simulink model "BlockModel"  (R2018b)
settings: Solver=ode45  StartTime=0.0  StopTime=10.0  RelTol=1e-3  EnableMultiTasking=on
PreLoadFcn:
  | load Buses
libraries: CustomLibrary x3
settings Model: Creator=Rose  LastModifiedBy=Rose
settings DataIOCC: LimitDataPoints=on  SaveFormat=Array  SignalLoggingSaveFormat=ModelDataLogs
settings OptimizationCC: DefaultParameterBehavior=Inlined  ExpressionDepthLimit=2147483647  LifeSpan=inf
settings DebuggingCC: UnderspecifiedInitializationDetection=Classic  MergeDetectMultiDrivingBlocksExec=none  SolverPrmCheckMsg=warning  FcnCallInpInsideContextMsg=warning  AllowSymbolicDim=off  StateNameClashWarn=warning  LibraryContextMissingDiagnostic=none  SFUnexpectedBacktrackingDiag=warning  SFNoUnconditionalDefaultTransitionDiag=warning  SFExecutionAtInitializationDiag=none
settings HardwareCC: ProdBitPerPointer=32  ProdBitPerSizeT=32  ProdBitPerPtrDiffT=32  ProdLargestAtomicFloat=None  ProdIntDivRoundTo=Undefined  ProdEndianess=Unspecified  ProdWordSize=32  ProdHWDeviceType=32-bit Generic
settings ModelReferenceCC: PropagateSignalLabelsOutOfModel=off
settings SFSimCC: SimUseLocalCustomCode=off
settings RTWCC: RTWUseLocalCustomCode=off
settings CodeAppCC: StateflowObjectComments=on
settings GRTTargetCC: TargetLangStandard=C89/C90 (ANSI)  GeneratePreprocessorConditionals=Disable all  CombineOutputUpdateFcns=off  GRTInterface=on
settings ConfigComp: CovMetricSettings=dw  CovHtmlReporting=on  CovSaveCumulativeToWorkspaceVar=on  CovSaveSingleToWorkspaceVar=on  CovExternalEMLEnable=off

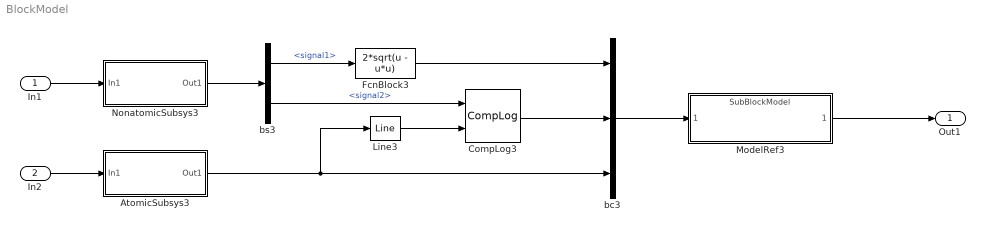
== system BlockModel ==
  In1 : Inport  OutDataTypeStr=Bus: Bus_2
  In2 : Inport  Port=2  OutDataTypeStr=int32  SampleTime=[0,1]
  AtomicSubsys3 : Subsystem  TreatAsAtomicUnit=on
  CompLog3 : CustomLibrary/CompLog  SystemSampleTime=-1
  FcnBlock3 : Fcn  Expr=2*sqrt(u - u*u)
  Line3 : CustomLibrary/Line  m=3  b=-1
  ModelRef3 : ModelReference  ModelNameDialog=SubBlockModel  SimulationMode=Normal  ModelReferenceVersion=1.41
  NonatomicSubsys3 : Subsystem
  bc3 : BusCreator  Inputs=3  OutDataTypeStr=Bus: Bus_2
  bs3 : BusSelector  OutputSignals=signal1,signal2
  Out1 : Outport  OutDataTypeStr=Bus: Bus_1
  wires:
  In1/1 -> NonatomicSubsys3/1(In1)
  In2/1 -> AtomicSubsys3/1(In1)
  NonatomicSubsys3/1(Out1) -> bs3/1
  bc3/1 -> ModelRef3/1
  AtomicSubsys3/1(Out1) -> Line3/1, bc3/3
  bs3/1 -> FcnBlock3/1  "<signal1>"
  bs3/2 -> CompLog3/1  "<signal2>"
  FcnBlock3/1 -> bc3/1
  CompLog3/1 -> bc3/2
  Line3/1 -> CompLog3/2
  ModelRef3/1 -> Out1/1

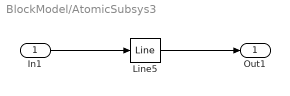
== system BlockModel/AtomicSubsys3 ==
  In1 : Inport  OutDataTypeStr=int32
  Line5 : CustomLibrary/Line  m=4  b=-1
  Out1 : Outport  OutDataTypeStr=int32
  wires:
  In1/1 -> Line5/1
  Line5/1 -> Out1/1

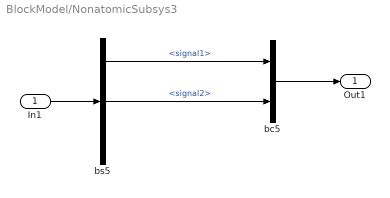
== system BlockModel/NonatomicSubsys3 ==
  In1 : Inport  OutDataTypeStr=Bus: Bus_2
  bc5 : BusCreator  Inputs=2  OutDataTypeStr=Bus: Bus_1
  bs5 : BusSelector  OutputSignals=signal1,signal2,signal3
  Out1 : Outport  OutDataTypeStr=Bus: Bus_1
  wires:
  In1/1 -> bs5/1
  bc5/1 -> Out1/1
  bs5/1 -> bc5/1  "<signal1>"
  bs5/2 -> bc5/2  "<signal2>"
